simulink library "PMV_PPD"  (R2013b)
settings: Solver=ode45  StartTime=0.0  StopTime=10.0  RelTol=1e-3
undefined symbols (not defined in the file): CarnotCallbacks_PMV_PPD
settings Model: Creator=drhf  LastModifiedBy=drhf

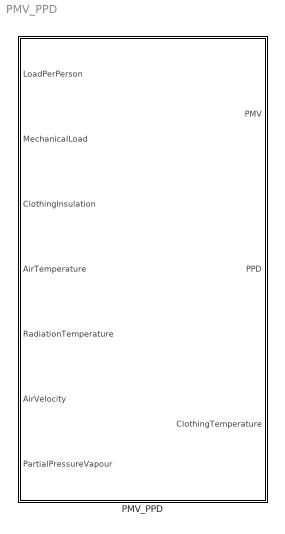
== system PMV_PPD ==
  PMV_PPD : Subsystem  LoadFcn=CarnotCallbacks_PMV_PPD('LoadFcn', gcb);  mask(PMV_PPD){DEBUGLEVEL=WARNINGLEVEL, MAXTOTALWARNINGS=inf, MAXCONSECUTIVEWARNINGS=inf, WRITETOFILE=0, FILENAME='messages.txt'}
      mask prompts: DEBUGLEVEL "Debug level"; MAXTOTALWARNINGS "maximum number of total warning"; MAXCONSECUTIVEWARNINGS "maximum number of consecutive warnings"; WRITETOFILE "write messages to file"; FILENAME "filename for messages"
      mask help: This block calculates from it's inputs the thermal comfort according to PMV (pedicted mean vote) and PPD (predicted percentage of dissatisfied).
      mask init:
      | %global debug level
      | [DEBUGLEVEL, MAXTOTALWARNINGS, MAXCONSECUTIVEWARNINGS, WRITETOFILE, FILENAME] = CarnotCallbacks_PMV_PPD('CheckDebugLevels', DEBUGLEVEL, MAXTOTALWARNINGS, MAXCONSECUTIVEWARNINGS, WRITETOFILE, FILENAME);
      mask TypeOptions DEBUGLEVEL: DEBUGLEVEL | INFOLEVEL | WARNINGLEVEL | ERRORLEVEL | FATALLEVEL | NOLEVEL
      mask Callback DEBUGLEVEL: CarnotCallbacks_PMV_PPD('MaskVisibilities');

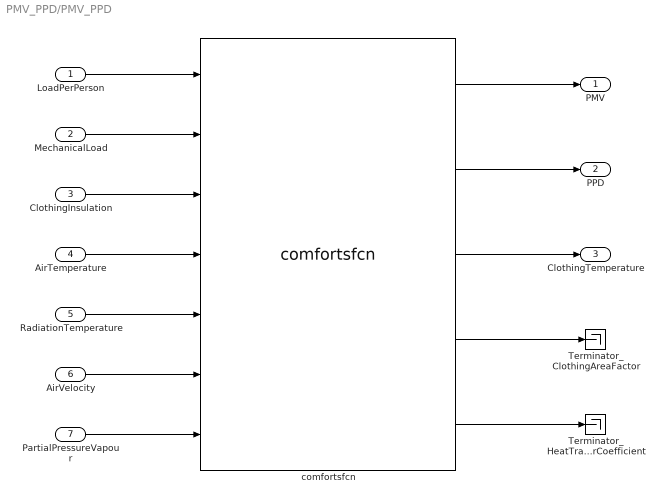
== system PMV_PPD/PMV_PPD ==
  LoadPerPerson : Inport
  MechanicalLoad : Inport  Port=2
  ClothingInsulation : Inport  Port=3
  AirTemperature : Inport  Port=4
  RadiationTemperature : Inport  Port=5
  AirVelocity : Inport  Port=6
  PartialPressureVapour : Inport  Port=7
  Terminator_ClothingAreaFactor : Terminator
  Terminator_HeatTransferCoefficient : Terminator
  comfortsfcn : S-Function  FunctionName=comfortsfcn  Parameters=DEBUGLEVEL-1, MAXTOTALWARNINGS, MAXCONSECUTIVEWARNINGS, WRITETOFILE, FILENAME  EnableBusSupport=off
  PMV : Outport
  PPD : Outport  Port=2
  ClothingTemperature : Outport  Port=3
  wires:
  PartialPressureVapour/1 -> comfortsfcn/7
  AirTemperature/1 -> comfortsfcn/4
  LoadPerPerson/1 -> comfortsfcn/1
  MechanicalLoad/1 -> comfortsfcn/2
  ClothingInsulation/1 -> comfortsfcn/3
  RadiationTemperature/1 -> comfortsfcn/5
  AirVelocity/1 -> comfortsfcn/6
  comfortsfcn/1 -> PMV/1
  comfortsfcn/2 -> PPD/1
  comfortsfcn/3 -> ClothingTemperature/1
  comfortsfcn/4 -> Terminator_ClothingAreaFactor/1
  comfortsfcn/5 -> Terminator_HeatTransferCoefficient/1
